simulink library "uavsimBlockset_ComputeNz"  (Simulink 8.0)
settings: Solver=ode45  StartTime=0.0  StopTime=10.0  RelTol=1e-3
libraries: aerolibtransform2 x1, dspmtrx3 x1
settings Model: Creator=mstolle  LastModifiedBy=j.bolting

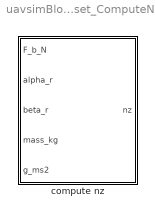
== system uavsimBlockset_ComputeNz ==
  compute nz : Subsystem

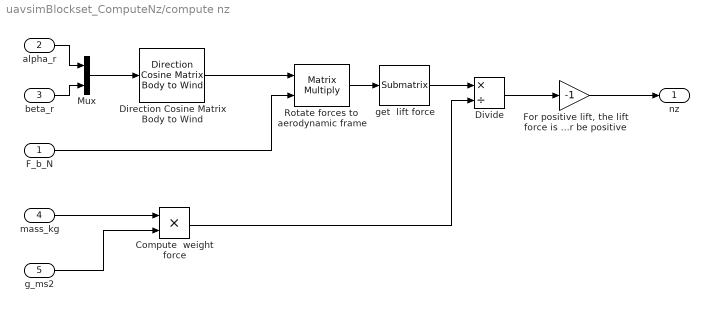
== system uavsimBlockset_ComputeNz/compute nz ==
  F_b_N : Inport
  alpha_r : Inport  Port=2
  beta_r : Inport  Port=3
  mass_kg : Inport  Port=4
  g_ms2 : Inport  Port=5
  Compute  weight force : Product  RndMeth=Zero
  Direction Cosine Matrix Body to Wind : aerolibtransform2/Direction Cosine Matrix Body to Wind
  Divide : Product  Inputs=*/
  "For positive lift, the lift force is negative due to the body frame's z axis pointing down (in cruise flight), the  load factor nz should however be positive" : Gain  Gain=-1
  Mux : Mux  Inputs=2
  Rotate forces to  aerodynamic frame : Product  Multiplication=Matrix(*)
  get  lift force : dspmtrx3/Submatrix  RowSpan=Range of rows  RowStartMode=Index  RowStartIndex=3  RowEndMode=Index  RowEndIndex=3  ColSpan=Range of columns  ColStartMode=First  ColStartIndex=1  ColEndMode=Last  ColEndIndex=1
  nz : Outport
  wires:
  "For positive lift, the lift force is negative due to the body frame's z axis pointing down (in cruise flight), the  load factor nz should however be positive"/1 -> nz/1
  beta_r/1 -> Mux/2
  alpha_r/1 -> Mux/1
  Mux/1 -> Direction Cosine Matrix Body to Wind/1
  Direction Cosine Matrix Body to Wind/1 -> Rotate forces to  aerodynamic frame/1
  F_b_N/1 -> Rotate forces to  aerodynamic frame/2
  Rotate forces to  aerodynamic frame/1 -> get  lift force/1
  get  lift force/1 -> Divide/1
  g_ms2/1 -> Compute  weight force/2
  mass_kg/1 -> Compute  weight force/1
  Compute  weight force/1 -> Divide/2
  Divide/1 -> "For positive lift, the lift force is negative due to the body frame's z axis pointing down (in cruise flight), the  load factor nz should however be positive"/1
